simulink model "bounding_box_calc"  (R2018a)
settings: Solver=VariableStepAuto  StartTime=0.0  StopTime=120  FixedStep=0.01  MaxStep=.001  RelTol=1e-3
settings Model: Creator=U500304  LastModifiedBy=Rafael
settings SolverCC: ZeroCrossAlgorithm=Adaptive
settings DataIOCC: SaveOutput=off  SaveTime=off
settings DebuggingCC: MaxConsecutiveZCsMsg=warning

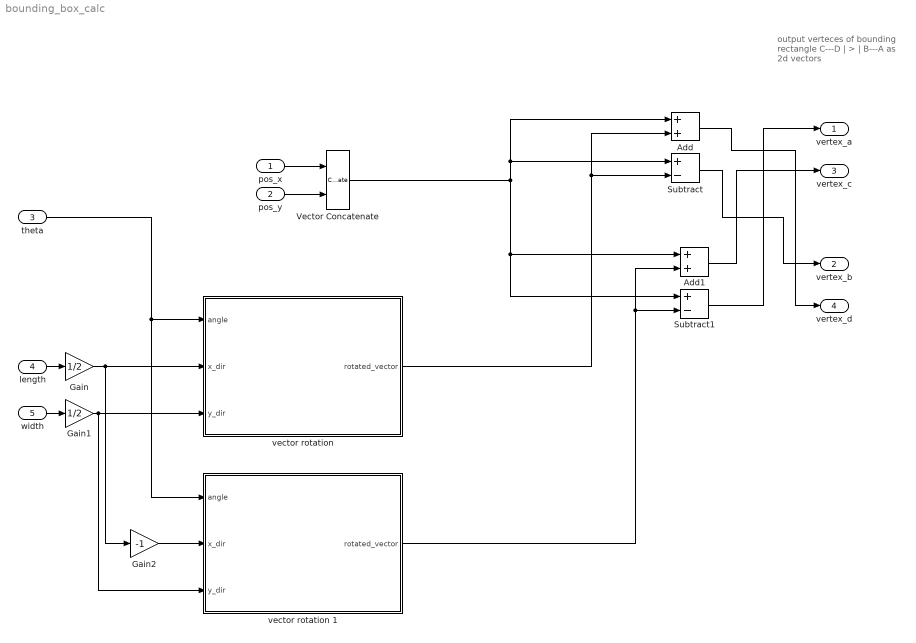
== system bounding_box_calc ==
  note: output verteces of
      | bounding rectangle
      | C---D
      | |  >  |
      | B---A  as 2d vectors
  pos_x : Inport  OutDataTypeStr=double  PortDimensions=1  SampleTime=0
  pos_y : Inport  Port=2  OutDataTypeStr=double  PortDimensions=1  SampleTime=0
  theta : Inport  Port=3  OutDataTypeStr=double  PortDimensions=1  SampleTime=0
  length : Inport  Port=4  OutDataTypeStr=double  PortDimensions=1
  width : Inport  Port=5  OutDataTypeStr=double  PortDimensions=1
  Add : Sum
  Add1 : Sum
  Gain : Gain  Gain=1/2
  Gain1 : Gain  Gain=1/2
  Gain2 : Gain  Gain=-1
  Subtract : Sum  Inputs=+-
  Subtract1 : Sum  Inputs=+-
  Vector Concatenate : Concatenate
  "vector rotation " : Subsystem
  vector rotation 1 : Subsystem
  vertex_a : Outport  OutDataTypeStr=double  PortDimensions=2  SampleTime=0
  vertex_b : Outport  Port=2  OutDataTypeStr=double  PortDimensions=2  SampleTime=0
  vertex_c : Outport  Port=3  OutDataTypeStr=double  PortDimensions=2  SampleTime=0
  vertex_d : Outport  Port=4  OutDataTypeStr=double  PortDimensions=2  SampleTime=0
  wires:
  Subtract/1 -> vertex_b/1
  Add1/1 -> vertex_c/1
  Add/1 -> vertex_d/1
  Subtract1/1 -> vertex_a/1
  width/1 -> Gain1/1
  length/1 -> Gain/1
  pos_x/1 -> Vector Concatenate/1
  pos_y/1 -> Vector Concatenate/2
  theta/1 -> "vector rotation "/1(angle), vector rotation 1/1(angle)
  Gain/1 -> "vector rotation "/2(x_dir), Gain2/1
  Gain2/1 -> vector rotation 1/2(x_dir)
  Gain1/1 -> "vector rotation "/3(y_dir), vector rotation 1/3(y_dir)
  Vector Concatenate/1 -> Add/1, Subtract/1, Add1/1, Subtract1/1
  "vector rotation "/1("rotated_vector ") -> Add/2, Subtract/2
  vector rotation 1/1("rotated_vector ") -> Add1/2, Subtract1/2

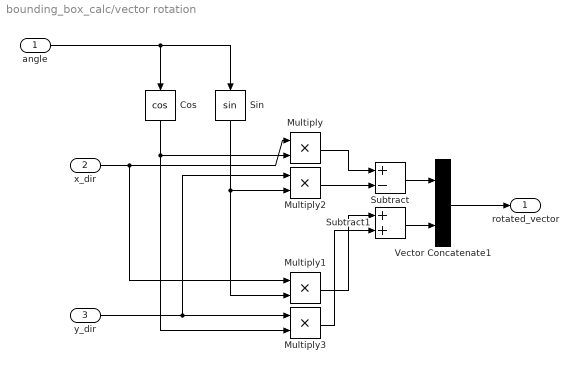
== system bounding_box_calc/vector rotation  ==
  angle : Inport
  x_dir : Inport  Port=2
  y_dir : Inport  Port=3
  Cos : Trigonometry  Operator=cos
  Multiply{,1..3} (4 alike) : Product
  Sin : Trigonometry
  Subtract : Sum  Inputs=+-
  Subtract1 : Sum
  Vector Concatenate1 : Concatenate
  "rotated_vector " : Outport
  wires:
  Multiply2/1 -> Subtract/2
  Subtract/1 -> Vector Concatenate1/1
  Vector Concatenate1/1 -> "rotated_vector "/1
  x_dir/1 -> Multiply/1, Multiply1/1
  angle/1 -> Sin/1, Cos/1
  Sin/1 -> Multiply2/2, Multiply1/2
  Cos/1 -> Multiply/2, Multiply3/2
  Subtract1/1 -> Vector Concatenate1/2
  y_dir/1 -> Multiply2/1, Multiply3/1
  Multiply/1 -> Subtract/1
  Multiply1/1 -> Subtract1/1
  Multiply3/1 -> Subtract1/2

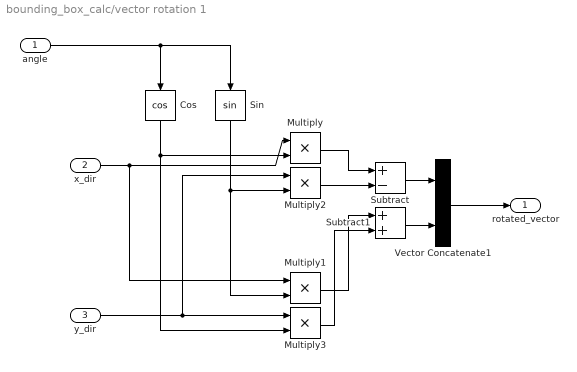
== system bounding_box_calc/vector rotation 1 ==
  angle : Inport
  x_dir : Inport  Port=2
  y_dir : Inport  Port=3
  Cos : Trigonometry  Operator=cos
  Multiply{,1..3} (4 alike) : Product
  Sin : Trigonometry
  Subtract : Sum  Inputs=+-
  Subtract1 : Sum
  Vector Concatenate1 : Concatenate
  "rotated_vector " : Outport
  wires:
  Multiply3/1 -> Subtract1/2
  Multiply1/1 -> Subtract1/1
  Multiply/1 -> Subtract/1
  y_dir/1 -> Multiply3/1, Multiply2/1
  Subtract1/1 -> Vector Concatenate1/2
  Cos/1 -> Multiply3/2, Multiply/2
  Sin/1 -> Multiply1/2, Multiply2/2
  angle/1 -> Cos/1, Sin/1
  x_dir/1 -> Multiply1/1, Multiply/1
  Vector Concatenate1/1 -> "rotated_vector "/1
  Subtract/1 -> Vector Concatenate1/1
  Multiply2/1 -> Subtract/2
